simulink model "carro"  (Simulink 7.7)
settings: Solver=ode45  StartTime=0.0  StopTime=stop_time  RelTol=1e-3
values from neighbouring files (symbols this model uses):
  beta = [10 25 50]    [Ex1.m]
  m = 50    [Ex1.m]
  v0 = [-1 +1]    [Ex1.m]
  y0 = 1    [Ex1.m]
undefined symbols (not defined in the file or in its folder): i
settings Model: Creator=g  LastModifiedBy=g
settings DebuggingCC: SolverPrmCheckMsg=none

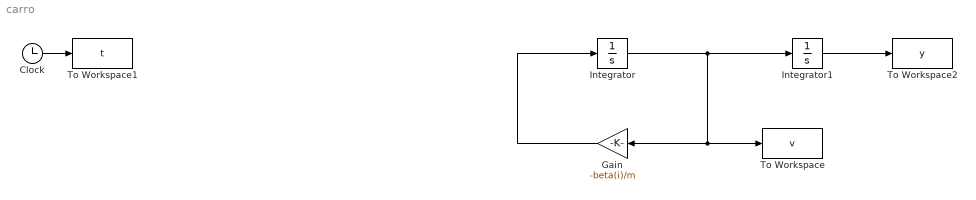
== system carro ==
  Clock : Clock
      settings: Decimation=10
  Gain : Gain  Gain=-beta(i)/m
  Integrator : Integrator  InitialCondition=v0
  Integrator1 : Integrator  InitialCondition=y0
  To Workspace : ToWorkspace  VariableName=v  SampleTime=-1  SaveFormat=Array
  To Workspace1 : ToWorkspace  VariableName=t  SampleTime=-1  SaveFormat=Array
  To Workspace2 : ToWorkspace  VariableName=y  SampleTime=-1  SaveFormat=Array
  wires:
  Integrator/1 -> Gain/1, To Workspace/1, Integrator1/1
  Gain/1 -> Integrator/1
  Clock/1 -> To Workspace1/1
  Integrator1/1 -> To Workspace2/1
